simulink subsystem "OdometriaHFz"  (R2024b)
settings: Solver=VariableStepAuto  StartTime=0.0  StopTime=10.0  RelTol=1e-3
undefined symbols (not defined in the file or in its folder): DiscIntNeverNeededParam
settings Model: Creator=Hajar  LastModifiedBy=Hajar
settings RTWCC: GPUComputeCapability=3.5

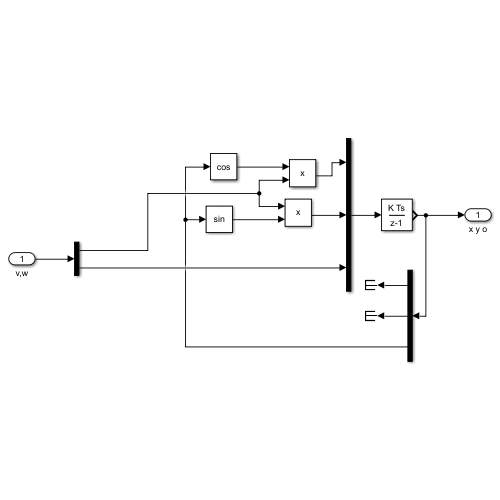
[thumbnail: Simulink's stored preview of the top-level diagram]
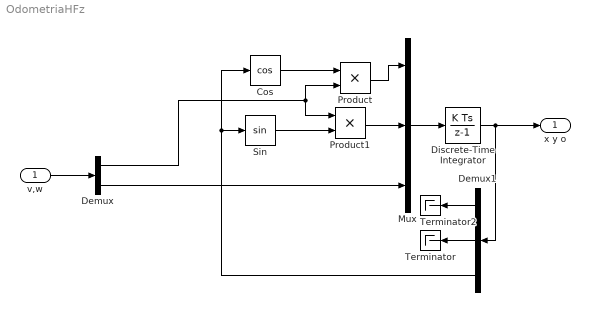
== system OdometriaHFz ==
  v,w : Inport
  Cos : Trigonometry  Operator=cos
  Demux : Demux  Outputs=2
  Demux1 : Demux  Outputs=3
  Discrete-Time Integrator : DiscreteIntegrator  SampleTime=-1  ICPrevOutput=DiscIntNeverNeededParam  ICPrevScaledInput=DiscIntNeverNeededParam
  Mux : Mux  Inputs=3
  Product : Product
  Product1 : Product
  Sin : Trigonometry
  Terminator : Terminator
  Terminator2 : Terminator
  x y o : Outport
  wires:
  v,w/1 -> Demux/1
  Cos/1 -> Product/1
  Sin/1 -> Product1/2
  Discrete-Time Integrator/1 -> x y o/1, Demux1/1
  Product/1 -> Mux/1
  Product1/1 -> Mux/2
  Demux/2 -> Mux/3
  Mux/1 -> Discrete-Time Integrator/1
  Demux1/1 -> Terminator2/1
  Demux1/3 -> Cos/1, Sin/1
  Demux1/2 -> Terminator/1
  Demux/1 -> Product1/1, Product/2
